simulink model "q3_a"  (R2026a)
settings: Solver=VariableStepAuto
model workspace (MAT data in the model file):
  T = Simulink.Parameter
  T.Value = 24
  T.Complexity = 'real'
  T.Dimensions = [1 1]
  T.DataType = 'auto'
settings Model: Creator=LAB_PC  LastModifiedBy=LAB_PC

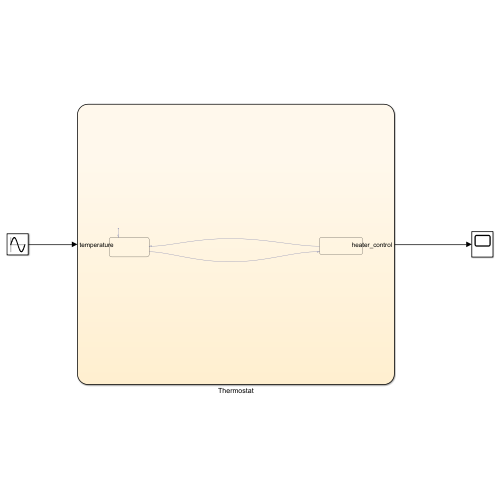
[thumbnail: Simulink's stored preview of the top-level diagram]
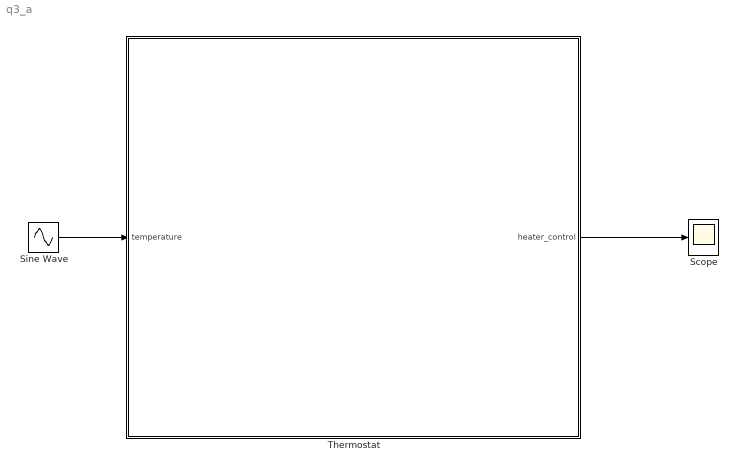
== system q3_a ==
  Scope : Scope
      settings: ActiveDisplayYMinimum=-7.2727900542120025  ActiveDisplayYMaximum=3.6285477534266057
  Sine Wave : Sin  Amplitude=5  Bias=24  SampleTime=0
  Thermostat : Stateflow chart  TreatAsAtomicUnit=on
  wires:
  Thermostat/1(heater_control) -> Scope/1
  Sine Wave/1 -> Thermostat/1(temperature)

== stateflow chart q3_a/Thermostat ==
  state Cooling
    entry:heater_control=0;
  state Heating
    entry: heater_control = 1;
  (default) -> Cooling
  Heating -> Cooling : [temperature > T]
  Cooling -> Heating : [temperature <T]
  data: heater_control output; temperature input; T parameter
